simulink model "ESE4481Simulink"  (R2024a)
settings: Solver=VariableStepAuto  StartTime=0.0  StopTime=10.0  RelTol=1e-3
undefined symbols (not defined in the file): aEval, bEval, fxc, fyc, Kp, Kphi, Kpn, Kpy, Kpz, Kq, Kr, Ktheta, Ku, Kv, Kw, Kyaw, mixMat, Pdc, Pec, Pnc, Yawc
settings Model: Creator=achic  LastModifiedBy=achic

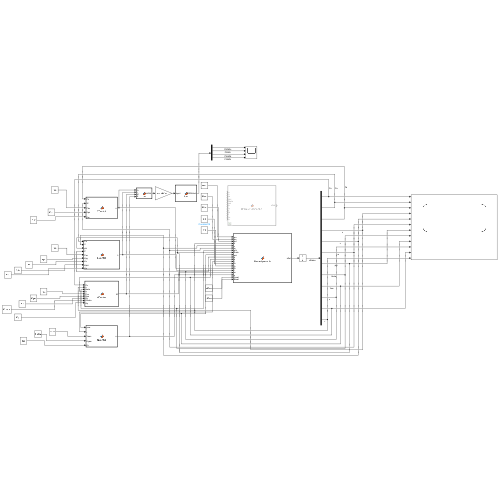
[thumbnail: Simulink's stored preview of the top-level diagram]
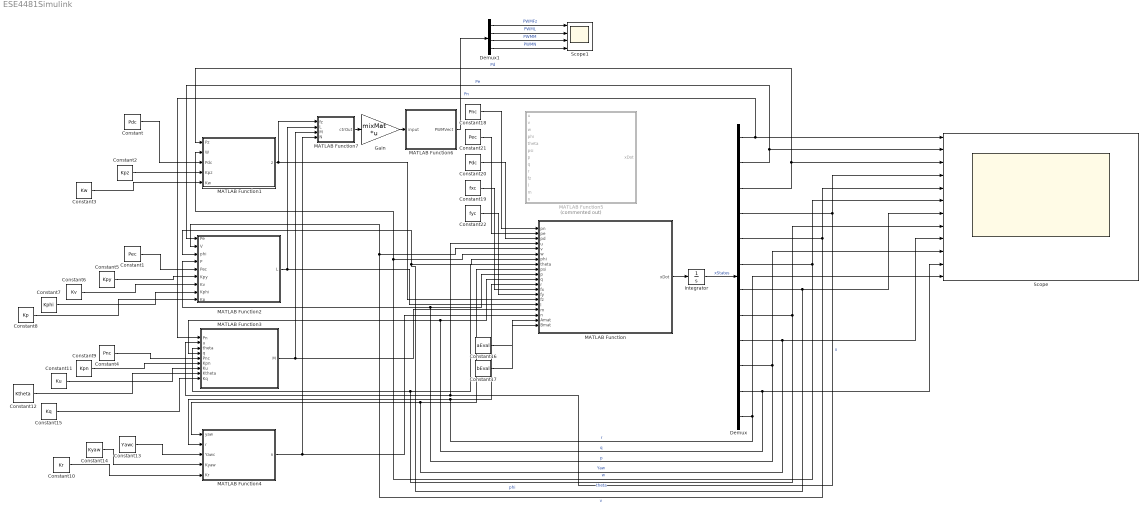
== system ESE4481Simulink ==
  Constant : Constant  Value=Pdc
  Constant1 : Constant  Value=Pec
  Constant10 : Constant  Value=Kr
  Constant11 : Constant  Value=Ku
  Constant12 : Constant  Value=Ktheta
  Constant13 : Constant  Value=Yawc
  Constant14 : Constant  Value=Kyaw
  Constant15 : Constant  Value=Kq
  Constant16 : Constant  Value=aEval
  Constant17 : Constant  Value=bEval
  Constant18 : Constant  Value=Pnc
  Constant19 : Constant  Value=fxc
  Constant2 : Constant  Value=Kpz
  Constant20 : Constant  Value=Pdc
  Constant21 : Constant  Value=Pec
  Constant22 : Constant  Value=fyc
  Constant3 : Constant  Value=Kw
  Constant4 : Constant  Value=Pnc
  Constant5 : Constant  Value=Kpy
  Constant6 : Constant  Value=Kv
  Constant7 : Constant  Value=Kphi
  Constant8 : Constant  Value=Kp
  Constant9 : Constant  Value=Kpn
  Demux : Demux  Outputs=12
  Demux1 : Demux
  Gain : Gain  Gain=mixMat  Multiplication=Matrix(K*u)
  Integrator : Integrator
  MATLAB Function : MATLAB Function  TreatAsAtomicUnit=on
  MATLAB Function1 : MATLAB Function  TreatAsAtomicUnit=on
  MATLAB Function2 : MATLAB Function  TreatAsAtomicUnit=on
  MATLAB Function3 : MATLAB Function  TreatAsAtomicUnit=on
  MATLAB Function4 : MATLAB Function  TreatAsAtomicUnit=on
  MATLAB Function5 : MATLAB Function  Commented=on  TreatAsAtomicUnit=on
  MATLAB Function6 : MATLAB Function  TreatAsAtomicUnit=on
  MATLAB Function7 : MATLAB Function  TreatAsAtomicUnit=on
  Scope : Scope  NumInputPorts=12
  Scope1 : Scope  NumInputPorts=4
  wires:
  MATLAB Function/1(xDot) -> Integrator/1
  Integrator/1 -> Demux/1  "xStates"
  Demux/4 -> MATLAB Function3/2(u), MATLAB Function/4(u), Scope/4  "u"
  Demux/5 -> Scope/5, MATLAB Function2/2(V), MATLAB Function/5(v)  "v"
  Demux/6 -> Scope/6, MATLAB Function1/2(W), MATLAB Function/6(w)  "w"
  Demux/7 -> Scope/7, MATLAB Function2/3(phi), MATLAB Function/7(phi)  "phi"
  Demux/8 -> Scope/8, MATLAB Function3/3(theta), MATLAB Function/8(theta)  "theta"
  Demux/9 -> Scope/9, MATLAB Function4/1(yaw), MATLAB Function/9(psi)  "Yaw"
  Demux/10 -> Scope/10, MATLAB Function/10(p), MATLAB Function2/4(P)  "p"
  Demux/11 -> Scope/11, MATLAB Function3/4(q), MATLAB Function/11(q)  "q"
  Demux/12 -> MATLAB Function4/2(r), MATLAB Function/12(r), Scope/12  "r"
  MATLAB Function1/1(z) -> MATLAB Function7/1(fz), MATLAB Function/15(fz)
  MATLAB Function2/1(L) -> MATLAB Function7/2(L), MATLAB Function/16(l)
  MATLAB Function3/1(M) -> MATLAB Function7/3(M), MATLAB Function/17(m)
  MATLAB Function4/1(n) -> MATLAB Function/18(n), MATLAB Function7/4(N)
  Constant2/1 -> MATLAB Function1/4(Kpz)
  Constant3/1 -> MATLAB Function1/5(Kw)
  Constant5/1 -> MATLAB Function2/6(Kpy)
  Constant6/1 -> MATLAB Function2/7(Kv)
  Constant7/1 -> MATLAB Function2/8(Kphi)
  Constant8/1 -> MATLAB Function2/9(Kp)
  Constant9/1 -> MATLAB Function3/6(Kpn)
  Constant11/1 -> MATLAB Function3/7(Ku)
  Constant12/1 -> MATLAB Function3/8(Ktheta)
  Constant14/1 -> MATLAB Function4/4(Kyaw)
  Constant10/1 -> MATLAB Function4/5(Kr)
  Demux/3 -> MATLAB Function1/1(Pz), Scope/3  "Pd"
  Demux/2 -> MATLAB Function2/1(Pe), Scope/2  "Pe"
  Demux/1 -> MATLAB Function3/1(Pn), Scope/1  "Pn"
  Constant15/1 -> MATLAB Function3/9(Kq)
  Constant16/1 -> MATLAB Function/19(Amat)
  Constant17/1 -> MATLAB Function/20(Bmat)
  Constant20/1 -> MATLAB Function/3(pd)
  Constant19/1 -> MATLAB Function/13(fx)
  Constant18/1 -> MATLAB Function/1(pn)
  Constant21/1 -> MATLAB Function/2(pe)
  Constant22/1 -> MATLAB Function/14(fy)
  MATLAB Function7/1(ctrOut) -> Gain/1
  Gain/1 -> MATLAB Function6/1(input)
  MATLAB Function6/1(PWMVect) -> Demux1/1
  Demux1/4 -> Scope1/4  "PWMN"
  Demux1/1 -> Scope1/1  "PWMFz"
  Demux1/2 -> Scope1/2  "PWML"
  Demux1/3 -> Scope1/3  "PWMM"
  Constant/1 -> MATLAB Function1/3(Pdc)
  Constant1/1 -> MATLAB Function2/5(Pec)
  Constant4/1 -> MATLAB Function3/5(Pnc)
  Constant13/1 -> MATLAB Function4/3(Yawc)

== matlab function ESE4481Simulink/MATLAB Function5 ==
  data: u input; xDot output; v input; w input; phi input; theta input; psi input; p input; q input; r input; fz input; l input; m input; n input
function xDot = DroneDynamNonLin(u, v, w, phi, theta, psi, p, q, r, fz, l, m, n)
    mass = 0.033; % Units = kg. Mass of drone.
    radius = 0.046; % the individual motor arm length (from motor stator to the drone’s
                    % center of gravity).
    g = 9.8; % m/s^2.

    cTheta = cosd(theta);
    cPhi = cosd(phi);
    cPsi = cosd(psi);
    
    sTheta = sind(theta);
    sPhi = sind(phi);
    sPsi = sind(psi);
    
    tTheta = tand(theta);
    
    
    
    %inerMatrix = Jy * eye(3); % Inertial Tensor matrix.
    inerMatrix = [16.57,  0.83,  0.72;
                   0.83, 16.66,  1.80;
                   0.72,  1.80, 29.26]; % Inertial Tensor matrix. In the body frame.
    
    Jx = inerMatrix(1, 1);
    Jxy = inerMatrix(2, 1);
    Jxz = inerMatrix(3, 1);
    %Jxy = inerMatrix(1, 2);
    Jy = inerMatrix(2, 2);
    Jyz = inerMatrix(3, 2);
    %Jxz = inerMatrix(1, 3);
    %Jyz = inerMatrix(2, 3);
    Jz = inerMatrix(3, 3);
    
    tau = Jx * Jz - Jxz^2;
    Tau1 = (Jxz * (Jx - Jy + Jz) ) / tau;
    Tau2 = (Jz * (Jz - Jy) + Jxz^2 ) / tau;
    Tau3 = Jz / tau;
    Tau4 = Jxz / tau;
    Tau5 = (Jz - Jx) / Jy;
    Tau6 = Jxz / Jy;
    Tau7 = ( (Jx - Jy) * Jx + Jxz^2) / tau;
    Tau8 = Jx / tau;
    % Creating the system of equations and putting it into a column vector.
    xDot = [(cTheta * cPsi) * u + (sPhi * sTheta * cPsi - cPhi * sPsi) * v + (cPhi * sTheta * cPsi + sPhi * sPsi)* w;
         (cTheta * sPsi) * u + (sPhi * sTheta * sPsi + cPhi * cPsi) * v + (cPhi * sTheta* sPsi - sPhi * cPsi) * w;
         (-sTheta) * u + (sPhi * cTheta) * v + (cPhi * cTheta) * w;
         r * v - q * w + fx / mass;
         p * w - r * u + fy / mass;
         q * u - p * v + fz / mass;
         p + (sPhi * tTheta) * q + (cPhi * tTheta) * r;
         0 + cPhi * q - sPhi * r;
         0 + (sPhi / cTheta) * q + (cPhi / cTheta) * r;
         (Tau1 * p * q - Tau2 * q * r) + Tau3 * l + Tau4 * n;
         Tau5 * p * r - Tau6 * (p^2 - r^2) + (1 / Jy) * m;
         Tau7 * p * q - Tau1 * q * r + Tau4 * l + Tau8 * n];
end

== matlab function ESE4481Simulink/MATLAB Function6 ==
  data: input input; PWMVect output
function PWMVect = fcn(input)

    fz = input(1);
    L = input(2);
    M = input(3);
    N = input(3);
    momentArmLeng = 0.046; % Units meters.
    
    PWMFromThrustFunc = @(thrust) (77371252455336267181195264 * sqrt(3296015354597325 * thrust / 38685626227668133590597632 + 182045336161068188949327330602267/178405961588244985132285746181186892047843328) / 3296015354597325 -  79924503786362355712/3296015354597325);
    
    PWMFromTorFunc = @(tor)  (19807040628566084398385987584 * sqrt(5032769273675311 * tor / 9903520314283042199192993792 + 663141903269232066005393670573721 / 23384026197294446691258957323460528314494920687616) /  5032769273675311 - 122038747880436514816 / 5032769273675311);

    LTorqForce = L / momentArmLeng; % Thrust force that makes torque L.
    MTorqForce = M / momentArmLeng;
    
    if fz < 0
        PWMFz = 0;
    else
        PWMFz = double(PWMFromThrustFunc(fz));
    end

    if L < 0
        PWML = 0;
    else 
        PWML = double(PWMFromThrustFunc(LTorqForce));
    end
    
    if M < 0
        PWMM = 0;
    else
        PWMM = double(PWMFromThrustFunc(MTorqForce));
    end

    if N < 0
        PWMN = 0;
    else
        PWMN = double(PWMFromTorFunc(N));
    end

    PWMVect = [PWMFz, PWML, PWMM, PWMN]';

end

== matlab function ESE4481Simulink/MATLAB Function7 ==
  data: fz input; ctrOut output; L input; M input; N input
function ctrOut = fcn(fz, L, M, N)
    
    
    ctrOut = [fz, L, M, N]';
end

== matlab function ESE4481Simulink/MATLAB Function1 ==
  data: Pz input; z output; W input; Pdc input; Kpz input; Kw input
function z = ZControl(Pz, W, Pdc, Kpz, Kw)
    % Using NED 
    K = [Pdc * Kpz * Kw, -Kpz * Kw, -Kw];
    stateVec = [1, Pz, W]';
    z = K * stateVec; 
end

== matlab function ESE4481Simulink/MATLAB Function ==
  data: pn input; pe input; pd input; u input; xDot output; v input; w input; phi input; theta input; psi input; p input; q input; r input; fx input; fy input; fz input; l input; m input; n input; Amat input; Bmat input
function xDot = DroneDynamLin(pn, pe, pd, u, v, w, phi, theta, psi, p, q, r, fx, fy, fz, l, m, n, Amat, Bmat)
    xVec = [pn, pe, pd, u, v, w, phi, theta, psi, p, q, r]';
    uVec = [fx, fy, fz, l, m, n]';
    xDot = Amat * xVec + Bmat * uVec;
end

== matlab function ESE4481Simulink/MATLAB Function2 ==
  data: L output; Pe input; V input; phi input; P input; Pec input; Kpy input; Kv input; Kphi input; Kp input
function L = LControl(Pe, V, phi, P, Pec, Kpy, Kv, Kphi, Kp)
    K = [Pec * Kpy * Kv * Kphi * Kp, -Kpy * Kv * Kphi * Kp, -Kv * Kphi * Kp, -Kphi * Kp, -Kp];
    stateVec = [1, Pe, V, phi, P]';
    L = K * stateVec; 
end

== matlab function ESE4481Simulink/MATLAB Function3 ==
  data: Pn input; u input; M output; theta input; q input; Pnc input; Kpn input; Ku input; Ktheta input; Kq input
function M = MControl(Pn, u, theta, q, Pnc, Kpn, Ku, Ktheta, Kq)
    K = [Pnc * Kpn * Ku * Ktheta * Kq, -Kpn *Ku * Ktheta * Kq, -Ku * Ktheta * Kq, -Ktheta * Kq, -Kq];
    stateVec = [1, Pn, u, theta, q]';
    M = K * stateVec; 
end

== matlab function ESE4481Simulink/MATLAB Function4 ==
  data: yaw input; n output; r input; Yawc input; Kyaw input; Kr input
function n = NControl(yaw, r, Yawc, Kyaw, Kr)
    K = [Yawc * Kyaw * Kr, -Kyaw * Kr, -Kr];
    stateVec = [1, yaw, r]';
    n = K * stateVec; 
end
